simulink model "pos_ctl_sim"  (R2023a)
settings: configuration reference "config" (kept outside this file)
model workspace (MATLAB code in the model file + MAT data in the model file):
  cmdLim = Simulink.Parameter
  cmdLim.Value = 15
  cmdLim.Description = 'Limit for controlling the maximum surface command angle.'
  cmdLim.Min = 0
  cmdLim.Max = 90
  cmdLim.DocUnits = 'deg'
  dispGain = Simulink.Parameter
  dispGain.Value = 0.75
  dispGain.Description = 'Gain applied to the displacement error.'
  dispGain.Min = 0
  dispGain.Max = []
  dispGain.DocUnits = 'deg/sec/deg'
  dispLim = Simulink.Parameter
  dispLim.Value = 30
  dispLim.Description = 'Limit for controlling the maximum commanded angle.'
  dispLim.Min = 0
  dispLim.Max = 180
  dispLim.DocUnits = 'deg'
  intGain = Simulink.Parameter
  intGain.Value = 0.5
  intGain.Description = 'Gain applied to the integral error.'
  intGain.Min = 0
  intGain.Max = []
  intGain.DocUnits = 'deg/sec/deg/sec'
  intLim = Simulink.Parameter
  intLim.Value = 5
  intLim.Description = 'Limit for controlling the maximum commanded angle.'
  intLim.Min = 0
  intLim.Max = 90
  intLim.DocUnits = 'deg'
  rateGain = Simulink.Parameter
  rateGain.Value = 2
  rateGain.Description = 'Gain applied to the rate error.'
  rateGain.Min = 0
  rateGain.Max = []
  rateGain.DocUnits = 'deg/deg/sec'
  rateLim = Simulink.Parameter
  rateLim.Value = 6
  rateLim.Description = 'Limit for controlling the maximum commanded angle.'
  rateLim.Min = 0
  rateLim.Max = 180
  rateLim.DocUnits = 'deg/sec'
  hdgGain = Simulink.Parameter
  hdgGain.Value = 0.015
  b = Simulink.Parameter
  b.Value = 0.001
  b.DataType = 'single'
  b.Complexity = 'real'
  b.Dimensions = [1 1]
  delta = Simulink.Parameter
  delta.Value = 6
  delta.Description = '电流环闭环带宽 rad/s'
  delta.DataType = 'single'
  delta.Complexity = 'real'
  delta.Dimensions = [1 1]
  enc_line = Simulink.Parameter
  enc_line.Value = 10000
  enc_line.DataType = 'single'
  enc_line.Complexity = 'real'
  enc_line.Dimensions = [1 1]
  enc_line_inv_p_n = Simulink.Parameter
  enc_line_inv_p_n.Value = 0.0001
  enc_line_inv_p_n.Description = '编码器分辨率 倒数'
  enc_line_inv_p_n.DataType = 'single'
  enc_line_inv_p_n.Complexity = 'real'
  enc_line_inv_p_n.Dimensions = [1 1]
  fc = Simulink.Parameter
  fc.Value = 0.001
  fc.DataType = 'single'
  fc.Complexity = 'real'
  fc.Dimensions = [1 1]
  flux = Simulink.Parameter
  flux.Value = 0.0125
  flux.DataType = 'single'
  flux.Complexity = 'real'
  flux.Dimensions = [1 1]
  fs = Simulink.Parameter
  fs.Value = 10000
  fs.Description = '位置环 速度环执行频率'
  fs.DataType = 'single'
  fs.Complexity = 'real'
  fs.Dimensions = [1 1]
  iq_max = Simulink.Parameter
  iq_max.Value = 10
  iq_max.DataType = 'single'
  iq_max.Complexity = 'real'
  iq_max.Dimensions = [1 1]
  j = Simulink.Parameter
  j.Value = 1.9e-05
  j.DataType = 'single'
  j.Complexity = 'real'
  j.Dimensions = [1 1]
  j_inv = Simulink.Parameter
  j_inv.Value = 52631.5789474
  j_inv.DataType = 'single'
  j_inv.Complexity = 'real'
  j_inv.Dimensions = [1 1]
  kt = Simulink.Parameter
  kt.Value = 0.075
  kt.DataType = 'single'
  kt.Complexity = 'real'
  kt.Dimensions = [1 1]
  ld = Simulink.Parameter
  ld.Value = 0.00059
  ld.Description = '定子电感 H'
  ld.DataType = 'single'
  ld.Complexity = 'real'
  ld.Dimensions = [1 1]
  ld_inv = Simulink.Parameter
  ld_inv.Value = 1694.91525424
  ld_inv.Description = '定子电感 H'
  ld_inv.DataType = 'single'
  ld_inv.Complexity = 'real'
  ld_inv.Dimensions = [1 1]
  lq = Simulink.Parameter
  lq.Value = 0.00059
  lq.Description = '定子电感 H'
  lq.DataType = 'single'
  lq.Complexity = 'real'
  lq.Dimensions = [1 1]
  lq_inv = Simulink.Parameter
  lq_inv.Value = 1694.91525424
  lq_inv.Description = '定子电感 H'
  lq_inv.DataType = 'single'
  lq_inv.Complexity = 'real'
  lq_inv.Dimensions = [1 1]
  pn = Simulink.Parameter
  pn.Value = 4
  pn.DataType = 'single'
  pn.Complexity = 'real'
  pn.Dimensions = [1 1]
  r = Simulink.Parameter
  r.Value = 1.02
  r.Description = '定子电阻 ohm'
  r.DataType = 'single'
  r.Complexity = 'real'
  r.Dimensions = [1 1]
  speed_obs_bw_hz = Simulink.Parameter
  speed_obs_bw_hz.Value = 800
  speed_obs_bw_hz.Description = '速度观测PLL带宽 HZ'
  speed_obs_bw_hz.DataType = 'single'
  speed_obs_bw_hz.Complexity = 'real'
  speed_obs_bw_hz.Dimensions = [1 1]
  tc = Simulink.Parameter
  tc.Value = 5e-05
  tc.Description = '电流环运行频率用来设定综合仿真的参数'
  tc.DataType = 'double'
  tc.Complexity = 'real'
  tc.Dimensions = [1 1]
  tp = Simulink.Parameter
  tp.Value = 0.0001
  tp.Description = '位置环速度环执行周期'
  tp.DataType = 'double'
  tp.Complexity = 'real'
  tp.Dimensions = [1 1]
  ts = Simulink.Parameter
  ts.Value = 1e-05
  ts.Description = '模型仿真的周期 s'
  ts.DataType = 'double'
  ts.Complexity = 'real'
  ts.Dimensions = [1 1]
  wn = Simulink.Parameter
  wn.Value = 6666.7
  wn.Description = '电流环闭环带宽 rad/s'
  wn.DataType = 'single'
  wn.Complexity = 'real'
  wn.Dimensions = [1 1]
settings Model: RequirementInfo={} %GIDa_fe9045fd_0412_4b6e_8206_617cc20e6fde  DataDictionary=model_config.sldd  ParameterArgumentNames=b,delta,enc_line,enc_line_inv_p_n,fc,flux,fs,iq_max,j,j_inv,kt,ld,ld_inv,lq,lq_inv,pn,r,speed_obs_bw_hz,wn  Creator=Administrator  LastModifiedBy=Administrator
settings ConfigSetRef: SourceName=config

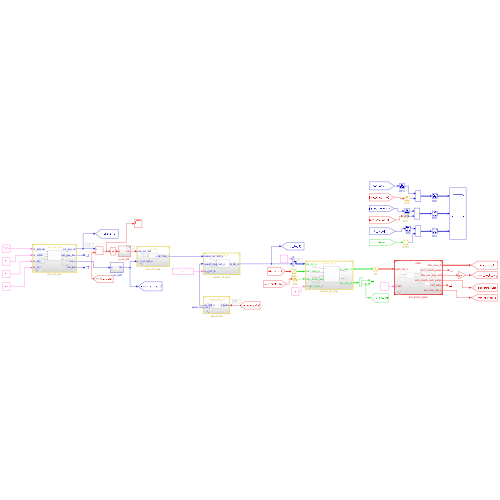
[thumbnail: Simulink's stored preview of the top-level diagram]
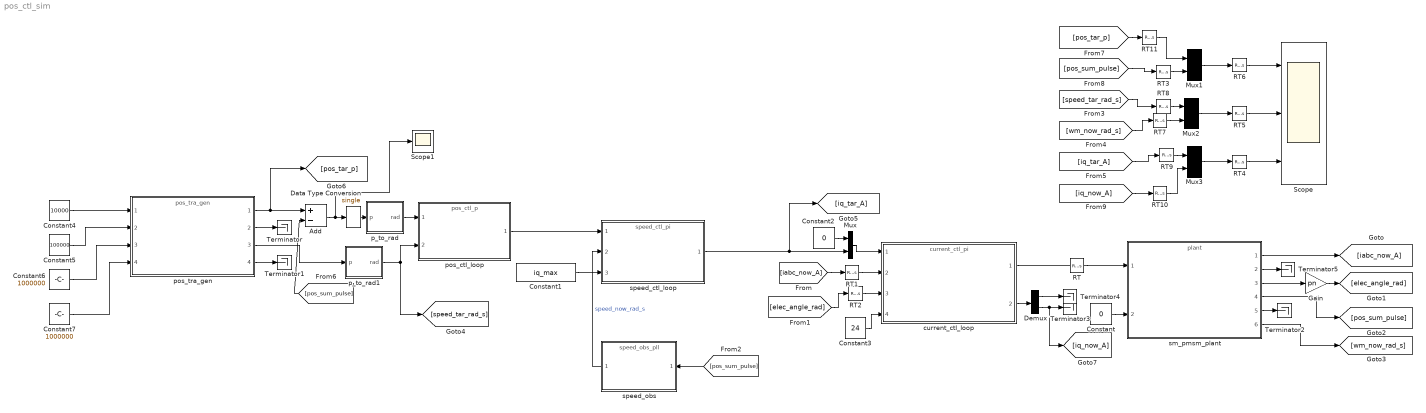
== system pos_ctl_sim ==
  Add : Sum  Inputs=+-
  Constant : Constant  Value=0  OutDataTypeStr=single
  Constant1 : Constant  Value=iq_max
  Constant2 : Constant  Value=0  OutDataTypeStr=single
  Constant3 : Constant  Value=24  OutDataTypeStr=single
  Constant4 : Constant  Value=10000  OutDataTypeStr=int64
  Constant5 : Constant  Value=100000  OutDataTypeStr=single
  Constant6 : Constant  Value=1000000  OutDataTypeStr=single
  Constant7 : Constant  Value=1000000  OutDataTypeStr=single
  Data Type Conversion : DataTypeConversion  OutDataTypeStr=single  SaturateOnIntegerOverflow=off  RndMeth=Floor
  Demux : Demux  Outputs=2
  Gain : Gain  Gain=pn
  Mux{,1..3} (4 alike) : Mux  Inputs=2
  RT : RateTransition  OutPortSampleTime=ts
  RT1 : RateTransition  OutPortSampleTime=tc
  RT{3..11} (9 alike) : RateTransition  OutPortSampleTime=tp
  RT2 : RateTransition  OutPortSampleTime=tc
  Scope : Scope  NumInputPorts=3
  Scope1 : Scope
  Terminator{,1..5} (6 alike) : Terminator
  current_ctl_loop : ModelReference  ModelNameDialog=current_ctl_pi.slx  UsingDefaultArgumentValue=0,0,0,0,0,0,0,0,0  SimulationMode=Normal  ModelReferenceVersion=2.138
  p_to_rad : Subsystem
  p_to_rad1 : Subsystem
  pos_ctl_loop : ModelReference  ModelNameDialog=pos_ctl_p.slx  UsingDefaultArgumentValue=0,0,0  SimulationMode=Normal  ModelReferenceVersion=2.45
  pos_tra_gen : ModelReference  ModelNameDialog=pos_tra_gen.slx  UsingDefaultArgumentValue=0  SimulationMode=Normal  ModelReferenceVersion=2.26
  sm_pmsm_plant : ModelReference  ModelNameDialog=plant.slx  UsingDefaultArgumentValue=0,0,0,0,0,0,0,0,0,0,0,0,0,0,0  SimulationMode=Normal  ModelReferenceVersion=1.23
  speed_ctl_loop : ModelReference  ModelNameDialog=speed_ctl_pi.slx  UsingDefaultArgumentValue=0,0,0,0  SimulationMode=Normal  ModelReferenceVersion=1.174
  speed_obs : ModelReference  ModelNameDialog=speed_obs_pll.slx  UsingDefaultArgumentValue=0,0,0  SimulationMode=Normal  ModelReferenceVersion=2.254
  wires:
  Constant/1 -> sm_pmsm_plant/2
  current_ctl_loop/1 -> RT/1
  sm_pmsm_plant/3 -> Gain/1
  sm_pmsm_plant/5 -> Terminator2/1
  RT/1 -> sm_pmsm_plant/1
  current_ctl_loop/2 -> Demux/1
  RT2/1 -> current_ctl_loop/3
  Demux/2 -> [iq_now_A], Terminator3/1
  RT1/1 -> current_ctl_loop/2
  Demux/1 -> Terminator4/1
  Constant3/1 -> current_ctl_loop/4
  sm_pmsm_plant/2 -> Terminator5/1
  pos_ctl_loop/1 -> speed_ctl_loop/1
  Constant1/1 -> speed_ctl_loop/3
  Constant2/1 -> Mux/1
  Mux/1 -> current_ctl_loop/1
  sm_pmsm_plant/1 -> [iabc_now_A]
  [iabc_now_A] -> RT1/1
  Gain/1 -> [elec_angle_rad]
  [elec_angle_rad] -> RT2/1
  sm_pmsm_plant/4 -> [pos_sum_pulse]
  sm_pmsm_plant/6 -> [wm_now_rad_s]
  speed_obs/1 -> speed_ctl_loop/2  "speed_now_rad_s"
  [pos_sum_pulse] -> speed_obs/1
  Add/1 -> Scope1/1, Data Type Conversion/1
  pos_tra_gen/1 -> [pos_tar_p], Add/1
  p_to_rad/1(rad) -> pos_ctl_loop/1
  p_to_rad1/1(rad) -> [speed_tar_rad_s], pos_ctl_loop/2
  pos_tra_gen/3 -> p_to_rad1/1(p)
  pos_tra_gen/2 -> Terminator/1
  pos_tra_gen/4 -> Terminator1/1
  Constant4/1 -> pos_tra_gen/1
  Constant5/1 -> pos_tra_gen/2
  Constant6/1 -> pos_tra_gen/3
  Constant7/1 -> pos_tra_gen/4
  [pos_sum_pulse] -> Add/2
  Data Type Conversion/1 -> p_to_rad/1(p)
  [pos_tar_p] -> RT11/1
  [pos_sum_pulse] -> RT3/1
  Mux1/1 -> RT6/1
  [speed_tar_rad_s] -> RT8/1
  [wm_now_rad_s] -> RT7/1
  Mux2/1 -> RT5/1
  [iq_tar_A] -> RT9/1
  [iq_now_A] -> RT10/1
  Mux3/1 -> RT4/1
  speed_ctl_loop/1 -> [iq_tar_A], Mux/2
  RT4/1 -> Scope/3
  RT5/1 -> Scope/2
  RT6/1 -> Scope/1
  RT3/1 -> Mux1/2
  RT7/1 -> Mux2/2
  RT8/1 -> Mux2/1
  RT9/1 -> Mux3/1
  RT10/1 -> Mux3/2
  RT11/1 -> Mux1/1

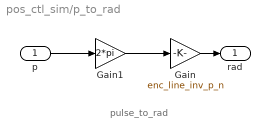
== system pos_ctl_sim/p_to_rad ==
  note: pulse_to_rad
  p : Inport
  Gain : Gain  Gain=enc_line_inv_p_n
  Gain1 : Gain  Gain=2*pi
  rad : Outport
  wires:
  p/1 -> Gain1/1
  Gain1/1 -> Gain/1
  Gain/1 -> rad/1

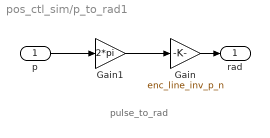
== system pos_ctl_sim/p_to_rad1 ==
  note: pulse_to_rad
  p : Inport
  Gain : Gain  Gain=enc_line_inv_p_n
  Gain1 : Gain  Gain=2*pi
  rad : Outport
  wires:
  Gain/1 -> rad/1
  Gain1/1 -> Gain/1
  p/1 -> Gain1/1
